simulink model "Three_Input_Model_CO"  (R2021a)
settings: Solver=VariableStepAuto  StartTime=0.0  StopTime=10  RelTol=1e-3
values from neighbouring files (symbols this model uses):
  A = double(subs(a,[x;u],equil))    [Funwork3_Main.m]    (also in Values.mat = [0 0 0 0 0 0 0 0 0 -8.175 65.4 -32.7 ... (36 elements, 6x6)]; Values_Rev2.mat = [0 0 0 0 0 0 0 0 0 -8.175 65.4 -32.7 ... (36 elements, 6x6)]; Values_Rev3.mat = [0 0 0 0 0 0 0 0 0 -0.534142885228 22.5045950602 -13.9882516)
  B = double(subs(b,[x;u],equil))    [Funwork3_Main.m]    (also in Values.mat = [0 0 0 0.666666666667 -1.33333333333 0]; Values_Rev2.mat = [0  0; 0  0; 0  0; 0.666666666667  -1.33333333333; -1.333333; Values_Rev3.mat = [0 0 0 0.425188099574 -0.174236211288 -0.288671680413 0 0 0 )
  C = [1 0 0 0 0 0 ... (first row only)    [Funwork3_Main.m]    (also in Values.mat = [1 0 0 0 1 0 0 0 1 0 0 0 ... (18 elements, 3x6)]; Values_Rev2.mat = [1 0 0 0 1 0 0 0 1 0 0 0 ... (18 elements, 3x6)]; Values_Rev3.mat = [1 0 0 0 1 0 0 0 1 0 0 0 ... (18 elements, 3x6)])
  K = M^-1*N    [Funwork3_Main.m]    (also in Values_Rev2.mat = [-2.68055786937  1.11424421179  -57.4156910728  -4.790622744; Values_Rev3.mat = [1104.07953515 279.420010905 157.104315976 182.686027553 129)
  L = P^-1*Y    [Funwork3_Main.m]    (also in Values_Rev2.mat = [4.4042 0 0 3.5453088 0 0 0 6.641 0 -8.175 75.26083176 -32.7; Values_Rev3.mat = [117.002054601 0.873440159496 -0.454542417964 4786.49521284 )
  u_e = zeros(3,1)    [Funwork3_Main.m]    (also in Values_Rev3.mat = [0 9.21172186389 3.90190360694])
  x0 = [0;-50*pi/180;-40*pi/180;0;0;0]    [Funwork3_Main.m]
  x_e = [0.1;theta1;theta2;0;0;0]    [Funwork3_Main.m]    (also in Values_Rev3.mat = [0.1 -1.0471975512 -0.785398163397 0 0 0])
libraries: vrlib x2, aerolibanimutils x1, dspvision x1
settings Model: Creator=J44381  LastModifiedBy=vicen
settings SolverCC: AlgebraicLoopSolver=TrustRegion
settings DebuggingCC: SFMachineParentedDataDiag=warning

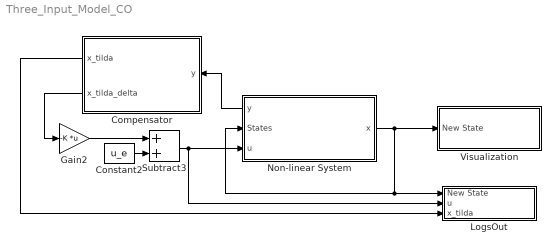
== system Three_Input_Model_CO ==
  Compensator : Subsystem
      settings: PortSchema="{\"entries\":[{\"content\":{\"sides\":[{\"content\":{\"connectorIds\":[\"Out1\",\"Out2\"]},\"type\":\"ConnectorPlacement.EquallySpacedRectSide\",\"uuid\":\"fa5a8305-86ae-432c-9810-dcf02cae709e\"},{\"content\":{\"connectorIds\":[\"In1\"],\"side\":\"RIGHT\"},\"type\":\"ConnectorPlacement.EquallySpacedRectSide\",\"uuid\":\"5b9e218f-8372-497e-90c9-36ba94e4ea20\"},{\"content\":{\"connectorIds\":[],\"side\":\"TOP\"},\"type\":\"ConnectorPlacement.EquallySpacedRectSide\",\"uuid\":\"bf766896-0790-4646-8f59-54f411e82d6d\"}]},\"type\":\"ConnectorPlacement.EquallySpacedConnector\",\"uuid\":\"810fb74e-5609-4dc4-a3e8-0485af32c7e5\"}],\"packageUris\":[\"http://schema.mathworks.com/mf0/Connector/R2020b\"],\"version\":\"1.0\"}"
  Constant2 : Constant  Value=u_e
  Gain2 : Gain  Gain=-K  Multiplication=Matrix(K*u)
  LogsOut : Subsystem
  Non-linear System : Subsystem
      settings: PortSchema="{\"entries\":[{\"content\":{\"sides\":[{\"content\":{\"connectorIds\":[\"Out2\",\"In1\",\"In2\"]},\"type\":\"ConnectorPlacement.EquallySpacedRectSide\",\"uuid\":\"e87e95e4-d445-42a4-8bb6-5db1cea140fd\"},{\"content\":{\"connectorIds\":[\"Out1\"],\"side\":\"RIGHT\"},\"type\":\"ConnectorPlacement.EquallySpacedRectSide\",\"uuid\":\"a4594086-6ae6-4dfa-940b-8e5ad9761096\"},{\"content\":{\"connectorIds\":[],\"side\":\"TOP\"},\"type\":\"ConnectorPlacement.EquallySpacedRectSide\",\"uuid\":\"2413b444-6401-41b3-9ef9-a53f71b4b630\"}]},\"type\":\"ConnectorPlacement.EquallySpacedConnector\",\"uuid\":\"ae149b85-3b76-4be2-80a6-ca3df1aa57f8\"}],\"packageUris\":[\"http://schema.mathworks.com/mf0/Connector/R2020b\"],\"version\":\"1.0\"}"
  Subtract3 : Sum
  Visualization : Subsystem
  wires:
  Non-linear System/1(x) -> Visualization/1(New State), LogsOut/1(New State), Non-linear System/1(States)
  Gain2/1 -> Subtract3/1
  Subtract3/1 -> Non-linear System/2(u), LogsOut/2(u)
  Constant2/1 -> Subtract3/2
  Compensator/1(x_tilda) -> LogsOut/3(x_tilda)
  Compensator/2(x_tilda_delta) -> Gain2/1
  Non-linear System/2(y) -> Compensator/1(y)

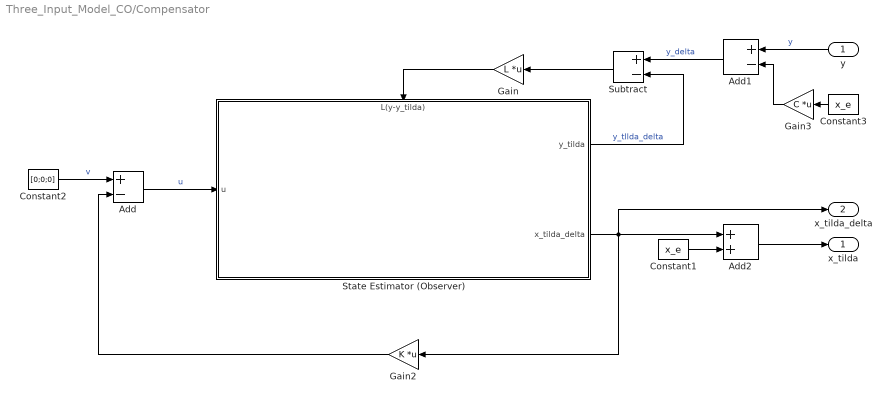
== system Three_Input_Model_CO/Compensator ==
  y : Inport
  Add : Sum  Inputs=+-
  Add1 : Sum  Inputs=+-
  Add2 : Sum
  Constant1 : Constant  Value=x_e
  Constant2 : Constant  Value=[0;0;0]
  Constant3 : Constant  Value=x_e
  Gain : Gain  Gain=L  Multiplication=Matrix(K*u)
  Gain2 : Gain  Gain=K  Multiplication=Matrix(K*u)
  Gain3 : Gain  Gain=C  Multiplication=Matrix(K*u)
  State Estimator (Observer) : Subsystem
      settings: PortSchema="{\"entries\":[{\"content\":{\"sides\":[{\"content\":{\"connectorIds\":[\"In1\"]},\"type\":\"ConnectorPlacement.EquallySpacedRectSide\",\"uuid\":\"af437ed9-8515-47ce-9bf3-57578eb1cf2e\"},{\"content\":{\"connectorIds\":[\"Out1\",\"Out2\"],\"side\":\"RIGHT\"},\"type\":\"ConnectorPlacement.EquallySpacedRectSide\",\"uuid\":\"1ea6d729-9487-4493-ae4f-2f3f5c430ca0\"},{\"content\":{\"connectorIds\":[\"In2\"],\"side\":\"TOP\"},\"type\":\"ConnectorPlacement.EquallySpacedRectSide\",\"uuid\":\"e9fc0f2c-a064-4175-9528-0d44140d355b\"}]},\"type\":\"ConnectorPlacement.EquallySpacedConnector\",\"uuid\":\"af498723-3483-4ae8-9449-73d3fe9ce68c\"}],\"packageUris\":[\"http://schema.mathworks.com/mf0/Connector/R2020b\"],\"version\":\"1.0\"}"
  Subtract : Sum  Inputs=+-
  x_tilda : Outport
  x_tilda_delta : Outport  Port=2
  wires:
  Add/1 -> State Estimator (Observer)/1(u)  "u"
  State Estimator (Observer)/1(y_tilda) -> Subtract/2  "y_tllda_delta"
  Subtract/1 -> Gain/1
  Constant2/1 -> Add/1  "v"
  State Estimator (Observer)/2(x_tilda_delta) -> Gain2/1, x_tilda_delta/1, Add2/1
  Gain/1 -> State Estimator (Observer)/2(L(y-y_tilda))
  Gain2/1 -> Add/2
  Constant1/1 -> Add2/2
  Add2/1 -> x_tilda/1
  Add1/1 -> Subtract/1  "y_delta"
  y/1 -> Add1/1  "y"
  Constant3/1 -> Gain3/1
  Gain3/1 -> Add1/2

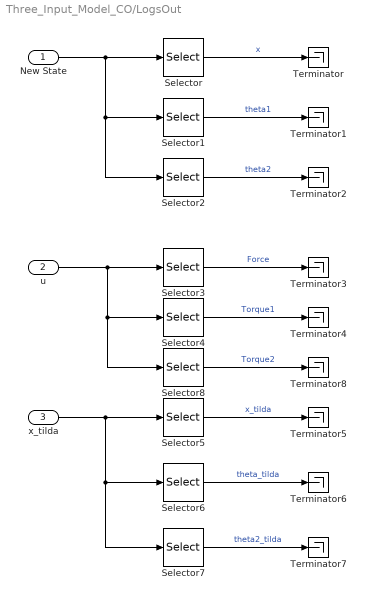
== system Three_Input_Model_CO/LogsOut ==
  New State : Inport
  u : Inport  Port=2
  x_tilda : Inport  Port=3
  Selector : Selector  InputPortWidth=6  IndexOptions=Index vector (dialog)  Indices=1  OutputSizes=1
  Selector1 : Selector  InputPortWidth=6  IndexOptions=Index vector (dialog)  Indices=2  OutputSizes=1
  Selector2 : Selector  InputPortWidth=6  IndexOptions=Index vector (dialog)  Indices=3  OutputSizes=1
  Selector3 : Selector  InputPortWidth=3  IndexOptions=Index vector (dialog)  Indices=1  OutputSizes=1
  Selector4 : Selector  InputPortWidth=3  IndexOptions=Index vector (dialog)  Indices=2  OutputSizes=1
  Selector5 : Selector  InputPortWidth=6  IndexOptions=Index vector (dialog)  Indices=1  OutputSizes=1
  Selector6 : Selector  InputPortWidth=6  IndexOptions=Index vector (dialog)  Indices=2  OutputSizes=1
  Selector7 : Selector  InputPortWidth=6  IndexOptions=Index vector (dialog)  Indices=3  OutputSizes=1
  Selector8 : Selector  InputPortWidth=3  IndexOptions=Index vector (dialog)  Indices=3  OutputSizes=1
  Terminator{,1..8} (9 alike) : Terminator
  wires:
  Selector/1 -> Terminator/1  "x"
  Selector1/1 -> Terminator1/1  "theta1"
  Selector2/1 -> Terminator2/1  "theta2"
  New State/1 -> Selector2/1, Selector1/1, Selector/1
  u/1 -> Selector8/1, Selector4/1, Selector3/1
  Selector4/1 -> Terminator4/1  "Torque1"
  Selector3/1 -> Terminator3/1  "Force"
  x_tilda/1 -> Selector5/1, Selector7/1, Selector6/1
  Selector5/1 -> Terminator5/1  "x_tilda"
  Selector6/1 -> Terminator6/1  "theta_tilda"
  Selector7/1 -> Terminator7/1  "theta2_tilda"
  Selector8/1 -> Terminator8/1  "Torque2"

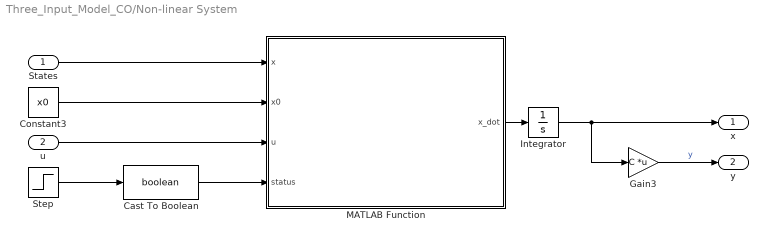
== system Three_Input_Model_CO/Non-linear System ==
  States : Inport
  u : Inport  Port=2
  Cast To Boolean : DataTypeConversion  OutDataTypeStr=boolean
  Constant3 : Constant  Value=x0  VectorParams1D=off  OutDataTypeStr=Bus: State_bus
  Gain3 : Gain  Gain=C  Multiplication=Matrix(K*u)
  Integrator : Integrator  InitialCondition=[x0.x;x0.theta1;x0.theta2;x0.x_dot;x0.theta1_dot;x0.theta2_dot]
  MATLAB Function : MATLAB Function  TreatAsAtomicUnit=on
  Step : Step  Time=.01  SampleTime=0
  x : Outport
  y : Outport  Port=2
  wires:
  MATLAB Function/1(x_dot) -> Integrator/1
  States/1 -> MATLAB Function/1(x)
  u/1 -> MATLAB Function/3(u)
  Step/1 -> Cast To Boolean/1
  Cast To Boolean/1 -> MATLAB Function/4(status)
  Gain3/1 -> y/1  "y"
  Integrator/1 -> Gain3/1, x/1
  Constant3/1 -> MATLAB Function/2(x0)

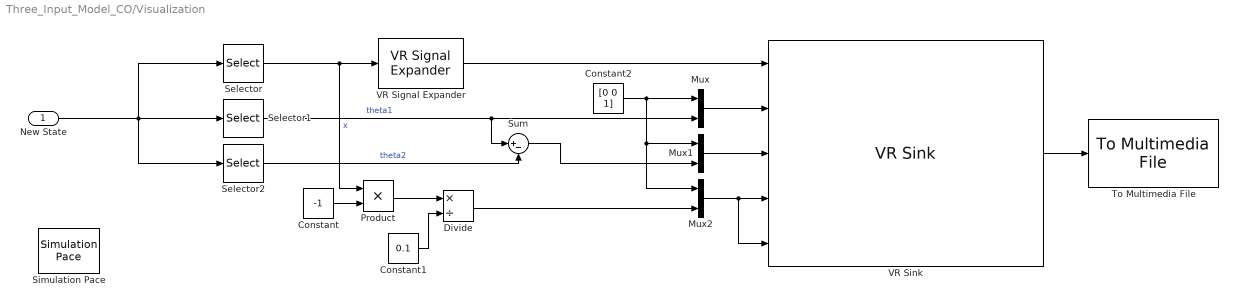
== system Three_Input_Model_CO/Visualization ==
  New State : Inport
  Constant : Constant  Value=-1
  Constant1 : Constant  Value=0.1
  Constant2 : Constant  Value=[0 0 1]
  Divide : Product  Inputs=*/
  Mux : Mux  Inputs=2
  Mux1 : Mux  Inputs=2
  Mux2 : Mux  Inputs=2
  Product : Product
  Selector : Selector  InputPortWidth=6  IndexOptions=Index vector (dialog)  Indices=1  OutputSizes=1
  Selector1 : Selector  InputPortWidth=6  IndexOptions=Index vector (dialog)  Indices=2  OutputSizes=1
  Selector2 : Selector  InputPortWidth=6  IndexOptions=Index vector (dialog)  Indices=3  OutputSizes=1
  Simulation Pace : aerolibanimutils/Simulation Pace  SimulationPace=1  SleepMode=Auto  OutputPaceError=off  SampleTime=1/30
  Sum : Sum  Inputs=|+-
  To Multimedia File : dspvision/To Multimedia File  outputFilename=output2.avi  streamSelection=Video only  videoCompressor=None (uncompressed)  audioCompressor=None (uncompressed)  imagePorts=One multidimensional signal  fileType=AVI  audioDatatype=Determine from input data type  fourcc=RGB  videoQuality=75  mj2000CompFactor=10
  VR Signal Expander : vrlib/VR Signal Expander  outwidth=3  outidx=[1]
  VR Sink : vrlib/VR Sink  InstantiateOnLoad=on  SampleTime=0.1  ViewEnable=on  RemoteChange=off  RemoteView=off  FieldsWritten=Cart.translation.3.1.1.double#Rotation1.rotation.4.1.1.double#Rotation2.rotation.4.1.1.double#Axis_Rotate.rotation.4.1.1.double#Axis_Rotate2.rotation.4.1.1.double  WorldFileName=Cart_Actual.WRL  AutoView=off  VideoDimensions=[1500 2000]  AllowVariableSize=off  FigureProperties="{'Position', 'Name', 'Viewpoint', 'CameraBound', 'CameraDirection', 'CameraPosition', 'CameraUpVector', 'ZoomFactor', 'Antialiasing', 'Headlight', 'Lighting', 'NavPanel', 'Sound', 'StatusBar', 'Stereo3D', 'Stereo3DCameraOffset', 'Stereo3DHIT', 'ToolBar', 'Textures', 'Transparency', 'Triad', 'Wireframe', 'NavZones', 'NavMode', 'NavSpeed', 'CaptureFileFormat', 'CaptureFileName', 'Record2DCompressMethod', 'Record2DCompressQuality', 'Record2D', 'Record2DFileName', 'Record2DFPS'; [1.2660000000000001e+02   9.4799999999999955e+01   8.0000000000000000e+02   6.0020000000000005e+02], '', '_untitled_1', 'on', [0.0000000000000000e+00   0.0000000000000000e+00  -1.0000000000000000e+00], [0.0000000000000000e+00   0.0000000000000000e+00   0.0000000000000000e+00], [0.0000000000000000e+00   1.0000000000000000e+00   0.0000000000000000e+00], [1.0000000000000000e+00], 'on', 'on', 'on', 'none', 'on', 'off', 'off', [1.0000000149011612e-01], [0.0000000000000000e+00], 'off', 'on', 'on', 'none', 'off', 'off', 'fly', 'normal', 'tif', '%f_anim_%n.tif', 'auto', [7.5000000000000000e+01], 'off', '***video***', 'auto'}"
  wires:
  New State/1 -> Selector/1, Selector2/1, Selector1/1
  Selector/1 -> VR Signal Expander/1, Product/1  "x"
  Selector1/1 -> Sum/1, Mux/2  "theta1"
  Product/1 -> Divide/1
  Constant/1 -> Product/2
  Constant1/1 -> Divide/2
  Constant2/1 -> Mux1/1, Mux2/1, Mux/1
  Selector2/1 -> Sum/2  "theta2"
  Divide/1 -> Mux2/2
  Sum/1 -> Mux1/2
  VR Signal Expander/1 -> VR Sink/1
  Mux/1 -> VR Sink/2
  Mux1/1 -> VR Sink/3
  Mux2/1 -> VR Sink/4, VR Sink/5
  VR Sink/1 -> To Multimedia File/1

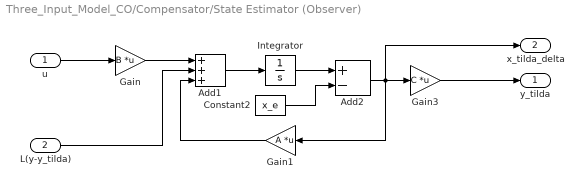
== system Three_Input_Model_CO/Compensator/State Estimator (Observer) ==
  u : Inport
  L(y-y_tilda) : Inport  Port=2
  Add1 : Sum  Inputs=+++
  Add2 : Sum  Inputs=+-
  Constant2 : Constant  Value=x_e
  Gain : Gain  Gain=B  Multiplication=Matrix(K*u)
  Gain1 : Gain  Gain=A  Multiplication=Matrix(K*u)
  Gain3 : Gain  Gain=C  Multiplication=Matrix(K*u)
  Integrator : Integrator  InitialCondition=[x0.x;0;0;x0.x_dot;x0.theta1_dot;x0.theta2_dot]
  y_tilda : Outport
  x_tilda_delta : Outport  Port=2
  wires:
  Gain1/1 -> Add1/3
  Add1/1 -> Integrator/1
  Gain/1 -> Add1/1
  u/1 -> Gain/1
  Gain3/1 -> y_tilda/1
  L(y-y_tilda)/1 -> Add1/2
  Constant2/1 -> Add2/2
  Add2/1 -> Gain3/1, Gain1/1, x_tilda_delta/1
  Integrator/1 -> Add2/1

== matlab function Three_Input_Model_CO/Non-linear System/MATLAB Function ==
  data: x input; x0 input; u input; x_dot output; status input
function x_dot  = Nonlinear_Dynamics(x,x0,u,status)
    if status == false
        x2 = x0.theta1;
        x3 = x0.theta2;
        x4 = x0.x_dot;
        x5 = x0.theta1_dot;
        x6 = x0.theta2_dot;
        u1 = u(1);
        u2 = u(2);
        u3 = u(3);
    else
        x2 = x(2);
        x3 = x(3);
        x4 = x(4);
        x5 = x(5);
        x6 = x(6);
        u1 = u(1);
        u2 = u(2);
        u3 = u(3);
    end
    % Insert Equations
    x_dot = double([
                     x4;
                     x5;
                     x6;
                     -(420*u1 - (2943*sin(2*x2))/2 + 150*x5^2*sin(x2) + (135*x6^2*sin(x3))/2 - 180*u1*cos(2*x2 - 2*x3) + 400*u3*cos(2*x2 - x3) - 840*u2*cos(x2) + 840*u3*cos(x2) - 400*u3*cos(x3) + (135*x6^2*sin(2*x2 - x3))/2 + 360*u2*cos(x2 - 2*x3) - 360*u3*cos(x2 - 2*x3))/(30*(5*cos(2*x2) + 9*cos(2*x2 - 2*x3) - 26));
                     (22800*u3 - 22800*u2 - 26487*sin(x2 - 2*x3) - 91233*sin(x2) + 3600*u2*cos(2*x3) - 3600*u3*cos(2*x3) + 4725*x6^2*sin(x2 - x3) + 750*x5^2*sin(2*x2) - 4000*u3*cos(x2 + x3) + 4200*u1*cos(x2) + 1350*x5^2*sin(2*x2 - 2*x3) - 1800*u1*cos(x2 - 2*x3) + 13600*u3*cos(x2 - x3) + 675*x6^2*sin(x2 + x3))/(150*(5*cos(2*x2) + 9*cos(2*x2 - 2*x3) - 26));
                     -(2700*sin(x2 - x3)*x5^2 + 1215*sin(2*x2 - 2*x3)*x6^2 + 13600*u3 - 26487*sin(2*x2 - x3) + 26487*sin(x3) - 4000*u3*cos(2*x2) + 1800*u1*cos(2*x2 - x3) + 3600*u2*cos(x2 + x3) - 3600*u3*cos(x2 + x3) - 1800*u1*cos(x3) - 12240*u2*cos(x2 - x3) + 12240*u3*cos(x2 - x3))/(135*(5*cos(2*x2) + 9*cos(2*x2 - 2*x3) - 26))
                ]);
            
end
